simulink subsystem "CasADi_freetf"  (R2024b)
settings: Solver=VariableStepAuto  StartTime=0.0  StopTime=10.0  RelTol=1e-3
undefined symbols (not defined in the file or in its folder): xf
settings Model: Creator=thatf  LastModifiedBy=thatf

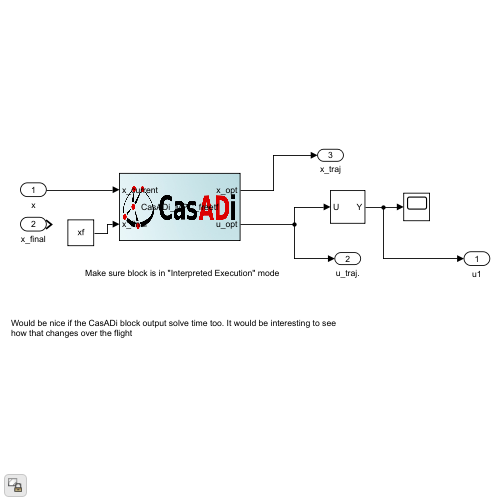
[thumbnail: Simulink's stored preview of the top-level diagram]
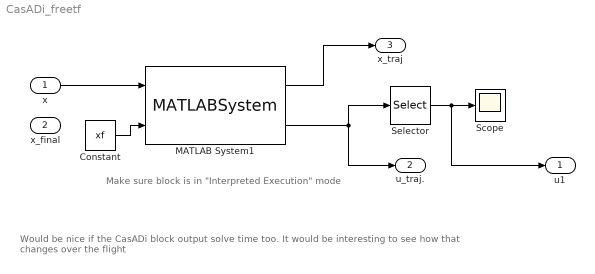
== system CasADi_freetf ==
  note: Make sure block is in "Interpreted Execution" mode
  note: Would be nice if the CasADi block output solve time too. It would be interesting to see how that changes over the flight
  x : Inport
  x_final : Inport  Port=2
  Constant : Constant  Value=xf
  MATLAB System1 : MATLABSystem  System=CasADi_MPC_freetf  vehicle=vehicle  steps=steps  max_iter=400  x_initial=x0  SimulateUsing=Interpreted execution  max_t_step=0.5  x_final=xf
      mask Type: CasADi_MPC_freetf
      mask Display:
      | image('CasADi.png');
      | disp('CasADi_MPC_freetf');
      | port_label('input',1,'x_current');
      | port_label('input',2,'x_final');
      | port_label('output',1,'x_opt');
      | port_label('output',2,'u_opt');
  Scope : Scope
  Selector : Selector  NumberOfDimensions=2  InputPortWidth=3  IndexOptions=Index vector (dialog),Select all  Indices=[1],1  OutputSizes=1,1
  u1 : Outport
  u_traj. : Outport  Port=2
  x_traj : Outport  Port=3
  wires:
  Selector/1 -> Scope/1, u1/1
  x/1 -> MATLAB System1/1
  MATLAB System1/1 -> x_traj/1
  MATLAB System1/2 -> u_traj./1, Selector/1
  Constant/1 -> MATLAB System1/2
